simulink model "generic_Truck_And_Trailer"  (R2025a)
settings: Solver=VariableStepAuto  StartTime=0.0  StopTime=350  FixedStep=0.01  MaxStep=0.001  RelTol=1e-3  EnableMultiTasking=on
libraries: TruckMaker4SL x250, simulink x1
(part 9 of 11)

== matlab function generic_Truck_And_Trailer/TruckMaker/Tractor_Subsystem /ONE_TRACK_MODEL_TRACTOR_UKF/MATLAB Function2 ==
  data: z input; u input; Q input; R input; Ts input; xhat output; data input; P output; dxdt output; innovation output; K_out output; S_out output; z_pred_out output
function [xhat, P, dxdt, innovation, K_out, S_out, z_pred_out] = UKF_OneTrack_IMU(z, u, Q, R, Ts, data)
z=z(1:5);
persistent x Pk dxdt_old t

%% =========================
%% INIT
%% =========================
if isempty(x)
    % [vx vy wz Cf Cr bax]
    x = [15;0.1;0.1;7.5;7.5;0];
end

if isempty(Pk)
    Pk = diag([0.1 0.1 0.1 5 5 0.5]);
end

if isempty(dxdt_old)
    dxdt_old = zeros(6,1);
end

if isempty(t)
    t = 0;
end

t = data;

if t < 30
    xhat = x;
    P = Pk;
    dxdt = dxdt_old;
    innovation = zeros(length(z),1);
    K_out = zeros(length(x), length(z));
    S_out = eye(length(z));
    z_pred_out = zeros(length(z),1);
    return
end

IDX_VX = 3;
IDX_VY = 4;

%% =========================
%% VEHICLE CONSTANTS
%% =========================
g  = 9.82;

p_cog = [3.473;0;0.925];
p_fax = [4.520;0;0.490];
p_rax = [0.950;0;0.490];
p_imu = [3.600;0;1.000];

lf = abs(p_fax(1)-p_cog(1));
lr = abs(p_cog(1)-p_rax(1));
L  = lf + lr;
h  = p_cog(3);

Rfax = p_fax - p_cog; Rfax(3) = -p_cog(3);
Rrax = p_rax - p_cog; Rrax(3) = -p_cog(3);
Rcog = p_imu - p_cog;

%% =========================
%% INPUTS
%% =========================
delta = u(1);
T_rl  = u(2);
T_rr  = u(3);
Rwheel = 0.505;
Fx_vehicle = (T_rl + T_rr)/Rwheel;

%% =========================
%% UKF PARAMS
%% =========================
n = length(x);
nSPx = 2*n + 1;

W0 = 1 - n/3;
Wi = (1 - W0)/(2*n);
gamma = sqrt(n/(1-W0));

%% =========================
%% SIGMA POINTS (PRIOR)
%% =========================
Pk = (Pk + Pk')/2 + 1e-9*eye(n);
Sx = chol(Pk,'lower');

X_pre = zeros(n,nSPx);
X_pre(:,1) = x;

for i=1:n
    X_pre(:,i+1)   = x + gamma*Sx(:,i);
    X_pre(:,i+1+n) = x - gamma*Sx(:,i);
end

%% =========================
%% PREDICTION
%% =========================
X_pred = zeros(n,nSPx);
dxdt_model = zeros(n,1);

m = 6800; 
Jz = 12994.917;

for k=1:nSPx

    Xk = X_pre(:,k);

    vx = Xk(1); vy = Xk(2); wz = Xk(3);
    Cf = Xk(4); Cr = Xk(5);
    bax = Xk(6);

    v_cog = [vx; vy; 0]; 
    omega = [0; 0; wz];

    Rotf = [cos(delta) -sin(delta) 0;
            sin(delta)  cos(delta) 0;
            0 0 1];

    vf = Rotf.'*(v_cog + cross(omega,Rfax));
    vr = v_cog + cross(omega,Rrax);

    alpha_f = atan2(vf(2), max(abs(vf(1)),0.1));
    alpha_r = atan2(vr(2), max(abs(vr(1)),0.1));

    ax_est = Fx_vehicle/m + vy*wz;

    Ffz = m*g*lr/L - m*ax_est*h/L;
    Frz = m*g*lf/L + m*ax_est*h/L;

    Fy_f = -Cf*alpha_f*Ffz;
    Fy_r = -Cr*alpha_r*Frz;

    dvx = (Fx_vehicle - Fy_f*sin(delta))/m + vy*wz + bax;

    % Testa DÄMPNING här (NYCKELN!)
    dvy = (Fy_f*cos(delta)+Fy_r)/m - vx*wz;

    dwz = (lf*Fy_f*cos(delta) - lr*Fy_r)/Jz;

    if k==1
        dxdt_model = [dvx; dvy; dwz; 0; 0; 0];
    end

    X_pred(:,k) = [
        vx + Ts*dvx
        vy + Ts*dvy
        wz + Ts*dwz
        Cf
        Cr
        bax
    ];
end

%% =========================
%% MEAN
%% =========================
x_pred = zeros(n,1);
for k=1:nSPx
    w = (k==1)*W0 + (k>1)*Wi;
    x_pred = x_pred + w*X_pred(:,k);
end

%% =========================
%% COVARIANCE
%% =========================
P_pred = zeros(n);
for k=1:nSPx
    w = (k==1)*W0 + (k>1)*Wi;
    dx = X_pred(:,k) - x_pred;
    P_pred = P_pred + w*(dx*dx');
end

P_pred = P_pred + Q*Ts;
P_pred = (P_pred + P_pred')/2 + 1e-9*eye(n);

%% =========================
%% SIGMA POINTS (POST)
%% =========================
Sx = chol(P_pred,'lower');

X_post = zeros(n,nSPx);
X_post(:,1) = x_pred;

for i=1:n
    X_post(:,i+1)   = x_pred + gamma*Sx(:,i);
    X_post(:,i+1+n) = x_pred - gamma*Sx(:,i);
end

%% =========================
%% MEASUREMENT MODEL
%% =========================
Z = zeros(length(z), nSPx);

for k=1:nSPx

    Xk = X_post(:,k);

    vx = Xk(1); vy = Xk(2); wz = Xk(3);
    Cf = Xk(4); Cr = Xk(5);
    bax = Xk(6);

    v_cog = [vx; vy; 0]; 
    omega=[0;0;wz];

    Rotf=[cos(delta) -sin(delta) 0;
          sin(delta)  cos(delta) 0;
          0 0 1];

    vf = Rotf.'*(v_cog+cross(omega,Rfax));
    vr = v_cog+cross(omega,Rrax);

    alpha_f = atan2(vf(2), max(abs(vf(1)),0.1));
    alpha_r = atan2(vr(2), max(abs(vr(1)),0.1));

    ax_est = Fx_vehicle/m + vy*wz;

    Ffz = m*g*lr/L - m*ax_est*h/L;
    Frz = m*g*lf/L + m*ax_est*h/L;

    Fy_f = -Cf*alpha_f*Ffz;
    Fy_r = -Cr*alpha_r*Frz;
    
    dvx = (Fx_vehicle - Fy_f*sin(delta))/m;
    dvy = (Fy_f*cos(delta)+Fy_r)/m;
    dwz = (lf*Fy_f*cos(delta) - lr*Fy_r)/Jz;

    a_cog = [dvx; dvy; 0];
    alpha_vec=[0;0;dwz];

    a_imu = a_cog + cross(omega,cross(omega,Rcog)) + cross(alpha_vec,Rcog);
    v_imu = v_cog + cross(omega,Rcog);

    ax_meas = a_imu(1) + bax;

    Z(:,k) = [
        ax_meas
        a_imu(2)
        v_imu(1:2)
        wz
    ];
end

%% =========================
%% MEASUREMENT MEAN
%% =========================
z_pred = zeros(length(z),1);
for k=1:nSPx
    w = (k==1)*W0 + (k>1)*Wi;
    z_pred = z_pred + w*Z(:,k);
end

%% =========================
%% SENSOR SELECTION
%% =========================
valid_idx = true(length(z),1);

if isnan(z(IDX_VX))
    valid_idx(IDX_VX) = false;
    valid_idx(IDX_VY) = false;
end

valid_idx = valid_idx & ~isnan(z);

z_used = z(valid_idx);
z_pred_used = z_pred(valid_idx);
Z_used = Z(valid_idx,:);
R_used = R(valid_idx,valid_idx);

%% =========================
%% S + Pxz
%% =========================
S_cov = zeros(length(z_used));
Pxz = zeros(n,length(z_used));

for k=1:nSPx
    w = (k==1)*W0 + (k>1)*Wi;

    dz = Z_used(:,k)-z_pred_used;
    dx = X_post(:,k)-x_pred;

    S_cov = S_cov + w*(dz*dz');
    Pxz = Pxz + w*(dx*dz');
end

S_cov = S_cov + R_used;
S_cov = (S_cov + S_cov')/2 + 1e-9*eye(size(S_cov));

%% =========================
%% UPDATE
%% =========================
K = Pxz / S_cov;

x = x_pred + K*(z_used - z_pred_used);
Pk = P_pred - K*S_cov*K';
Pk = (Pk + Pk')/2 + 1e-9*eye(n);

%% =========================
%% OUTPUT
%% =========================
xhat = x;
P = Pk;
dxdt = dxdt_model;

innovation = zeros(length(z),1);
innovation(valid_idx) = z_used - z_pred_used;

K_out = zeros(n,length(z));
K_out(:,valid_idx) = K;

S_out = zeros(length(z));
S_out(valid_idx,valid_idx) = S_cov;

z_pred_out = z_pred;

end

== matlab function generic_Truck_And_Trailer/TruckMaker/Tractor_Subsystem /ONE_TRACK_MODEL_TRACTOR_UKF/UKF_ONE_TRACK1 ==
  data: z input; u input; xhat output; Q input; R input; Ts input; P output; dxdt output; innovation output; K_out output; S_out output; z_pred_out output; data input
function [xhat, P, dxdt, innovation, K_out, S_out, z_pred_out] = UKF_OneTrack_IMU(z, u, Q, R, Ts,data)

persistent x Pk dxdt_old t p_nom Pp

if isempty(x)
    x = [15;0.1;0.1;7.5;7.5];
end
if isempty(Pk)
    Pk = diag([0.1 0.1 0.1 5 5]);
end
if isempty(dxdt_old)
    dxdt_old = zeros(5,1);
end
if isempty(t)
    t = 0;
end
if isempty(p_nom)
    p_nom = [6800; 12994.917];
    Pp = diag([5000, 20000]).^2;
end

T_sim = 0.001;
t = t + T_sim;
t=data;

if t < 30
    xhat = x;
    P = Pk;
    dxdt = dxdt_old;
    innovation = zeros(length(z),1);
    K_out = zeros(length(x), length(z));
    S_out = eye(length(z));
    z_pred_out = zeros(length(z),1);
    return
end

IDX_VX  = 3; 
IDX_WRL = 6; 
IDX_WRR = 7;

g  = 9.82;

p_cog = [3.473;0;0.925];
p_fax = [4.520;0;0.490];
p_rax = [0.950;0;0.490];
p_imu = [3.600;0;1.000];

lf = abs(p_fax(1)-p_cog(1));
lr = abs(p_cog(1)-p_rax(1));
L  = lf + lr;
h  = p_cog(3);

Rfax = p_fax - p_cog; Rfax(3) = -p_cog(3);
Rrax = p_rax - p_cog; Rrax(3) = -p_cog(3);
Rcog = p_imu - p_cog;

delta = u(1);
T_rl  = u(2);
T_rr  = u(3);
Rwheel = 0.505;
Fx_vehicle = (T_rl + T_rr)/Rwheel;

n  = length(x);
np = length(p_nom);
nSPx = 2*n + 1;
nSPp = 2*np;
nSP  = nSPx + nSPp;

W0 = 1 - (n + np)/3;
Wi = (1 - W0)/(2*(n + np));
gamma = sqrt((n + np)/(1 - W0));

%% ===== STATE SIGMA =====
Pk = (Pk + Pk')/2 + 1e-9*eye(n);
Sx = chol(Pk,'lower');

X = zeros(n,nSPx);
X(:,1) = x;
for i=1:n
    X(:,i+1)   = x + gamma*Sx(:,i);
    X(:,i+1+n) = x - gamma*Sx(:,i);
end

%% ===== PARAM SIGMA =====
Pp = (Pp + Pp')/2 + 1e-9*eye(np);
Sp = chol(Pp,'lower');

SPp = zeros(np,nSPp);
for i=1:np
    SPp(:,i)    = p_nom + gamma*Sp(:,i);
    SPp(:,i+np) = p_nom - gamma*Sp(:,i);
end

%% ===== PREDICTION =====
X_prop = zeros(n,nSP);
dxdt_model = zeros(5,1);

for k=1:nSP
    if k <= nSPx
        Xk = X(:,k); 
        pk = p_nom;
    else
        Xk = x; 
        pk = SPp(:,k-nSPx);
    end

    vx=Xk(1); vy=Xk(2); wz=Xk(3); Cf=Xk(4); Cr=Xk(5);
    m=pk(1); Jz=pk(2);

    v_cog=[vx;vy;0]; omega=[0;0;wz];
    Rotf=[cos(delta) -sin(delta) 0; sin(delta) cos(delta) 0; 0 0 1];

    vf=Rotf.'*(v_cog+cross(omega,Rfax));
    vr=v_cog+cross(omega,Rrax);

    alpha_f=atan2(vf(2),max(abs(vf(1)),0.1));
    alpha_r=atan2(vr(2),max(abs(vr(1)),0.1));

    ax_est=Fx_vehicle/m+vy*wz;

    Ffz=m*g*lr/L - m*ax_est*h/L;
    Frz=m*g*lf/L + m*ax_est*h/L;

    Fy_f=-Cf*alpha_f*Ffz;
    Fy_r=-Cr*alpha_r*Frz;

    dvx=(Fx_vehicle - Fy_f*sin(delta))/m + vy*wz;
    dvy=(Fy_f*cos(delta)+Fy_r)/m - vx*wz;
    dwz=(lf*Fy_f*cos(delta) - lr*Fy_r)/Jz;

    if k==1
        dxdt_model=[dvx;dvy;dwz;0;0];
    end

    X_prop(:,k)=[vx+Ts*dvx; vy+Ts*dvy; wz+Ts*dwz; Cf; Cr];
end

%% ===== MEAN =====
x_pred=zeros(n,1);
for k=1:nSP
    w=(k==1)*W0 + (k>1)*Wi;
    x_pred=x_pred + w*X_prop(:,k);
end

%% ===== COV =====
P_pred=zeros(n);
for k=1:nSPx
    w=(k==1)*W0 + (k>1)*Wi;
    dx=X_prop(:,k)-x_pred;
    P_pred=P_pred + w*(dx*dx');
end
P_pred=P_pred + Q*Ts;

%% ===== NEW SIGMA POINTS =====
P_pred=(P_pred+P_pred')/2 + 1e-9*eye(n);
Sx=chol(P_pred,'lower');

SPx_new=zeros(n,nSPx);
SPx_new(:,1)=x_pred;

for i=1:n
    SPx_new(:,i+1)=x_pred+gamma*Sx(:,i);
    SPx_new(:,i+1+n)=x_pred-gamma*Sx(:,i);
end

%% ===== MEASUREMENT =====
Z=zeros(length(z),nSP);

for k=1:nSP
    if k<=nSPx
        Xk=SPx_new(:,k);
        pk=p_nom;
    else
        Xk=x_pred;
        pk=SPp(:,k-nSPx);
    end

    vx=Xk(1); vy=Xk(2); wz=Xk(3);
    Cf=Xk(4); Cr=Xk(5);

    m=pk(1); Jz=pk(2);

    v_cog=[vx;vy;0]; omega=[0;0;wz];
    Rotf=[cos(delta) -sin(delta) 0; sin(delta) cos(delta) 0; 0 0 1];

    vf=Rotf.'*(v_cog+cross(omega,Rfax));
    vr=v_cog+cross(omega,Rrax);

    alpha_f=atan2(vf(2),max(abs(vf(1)),0.1));
    alpha_r=atan2(vr(2),max(abs(vr(1)),0.1));

    ax_est=Fx_vehicle/m+vy*wz;

    Ffz=m*g*lr/L - m*ax_est*h/L;
    Frz=m*g*lf/L + m*ax_est*h/L;

    Fy_f=-Cf*alpha_f*Ffz;
    Fy_r=-Cr*alpha_r*Frz;

    dvx=(Fx_vehicle - Fy_f*sin(delta))/m;
    dvy=(Fy_f*cos(delta)+Fy_r)/m;
    dwz=(lf*Fy_f*cos(delta) - lr*Fy_r)/Jz;

    a_cog=[dvx;dvy;0];
    alpha_vec=[0;0;dwz];

    a_imu=a_cog + cross(omega,cross(omega,Rcog)) + cross(alpha_vec,Rcog);
    v_imu=v_cog + cross(omega,Rcog);

    omega_rl=vx/Rwheel;
    omega_rr=vx/Rwheel;

    Z(:,k)=[a_imu(1:2); v_imu(1:2); wz; omega_rl; omega_rr];
end

%% ===== z mean =====
z_pred=zeros(length(z),1);
for k=1:nSP
    w=(k==1)*W0 + (k>1)*Wi;
    z_pred=z_pred + w*Z(:,k);
end

%% ===== SENSOR SELECTION =====
valid_idx=true(length(z),1);

if ~isnan(z(IDX_VX))
    valid_idx(IDX_WRL)=false;
    valid_idx(IDX_WRR)=false;
else
    valid_idx(IDX_VX)=false;
end

valid_idx=valid_idx & ~isnan(z);

z_used=z(valid_idx);
z_pred_used=z_pred(valid_idx);
Z_used=Z(valid_idx,:);
R_used=R(valid_idx,valid_idx);

%% ===== S =====
S_cov=zeros(length(z_used));
for k=1:nSP
    w=(k==1)*W0 + (k>1)*Wi;
    dz=Z_used(:,k)-z_pred_used;
    S_cov=S_cov + w*(dz*dz');
end

S_cov=S_cov + R_used;
S_cov=(S_cov+S_cov')/2 + 1e-9*eye(size(S_cov));

%% ===== Pxz =====
Pxz=zeros(n,length(z_used));
for k=1:nSPx
    w=(k==1)*W0 + (k>1)*Wi;
    dx=SPx_new(:,k)-x_pred;
    dz=Z_used(:,k)-z_pred_used;
    Pxz=Pxz + w*(dx*dz');
end

%% ===== UPDATE =====
K=Pxz/S_cov;

x=x_pred + K*(z_used - z_pred_used);
Pk=P_pred - K*S_cov*K';
Pk=(Pk+Pk')/2 + 1e-9*eye(n);

%% ===== OUTPUT =====
xhat=x;
P=Pk;
dxdt=dxdt_model;

innovation=zeros(length(z),1);
innovation(valid_idx)=z_used - z_pred_used;

K_out=zeros(n,length(z));
K_out(:,valid_idx)=K;

S_out=zeros(length(z));
S_out(valid_idx,valid_idx)=S_cov;

z_pred_out=z_pred;

end

== matlab function generic_Truck_And_Trailer/TruckMaker/Tractor_Subsystem /ONE_TRACK_MODEL_TRACTOR_UKF/Working Model with 5 measurements  ==
  data: z input; u input; xhat output; Q input; R input; Ts input; P output; dxdt output; innovation output; K_out output; S_out output; z_pred_out output
function [xhat, P, dxdt, innovation, K_out, S_out, z_pred_out] = UKF_OneTrack_IMU(z, u, Q, R, Ts)

% z = [ax; ay; vx; vy; wz]

%% =========================
%% PERSISTENT VARIABLES
%% =========================
persistent x Pk dxdt_old t

if isempty(x)
    x = [15;0.1;0.1;7.5;7.5];   % [vx vy wz Cf Cr]
end
if isempty(Pk)
    Pk = diag([0.1 0.1 0.1 2 2]);
end
if isempty(dxdt_old)
    dxdt_old = zeros(5,1);
end
if isempty(t)
    t = 0;
end

%% =========================
%% TIME UPDATE
%% =========================
t = t + 0.001;

start_time = 30;
if t < start_time
    xhat = x;
    P = Pk;
    dxdt = dxdt_old;

    innovation = zeros(length(z),1);
    K_out = zeros(length(x), length(z));
    S_out = eye(length(z));
    z_pred_out = zeros(length(z),1);
    return
end

%% =========================
%% VEHICLE PARAMETERS
%% =========================
m  = 6800;
g  = 9.82;
Jz = 12994.917;

p_cog = [3.473;0;0.925];
p_fax = [4.520;0;0.490];
p_rax = [0.950;0;0.490];
p_imu = [3.600;0;1.000];

lf = abs(p_fax(1)-p_cog(1));
lr = abs(p_cog(1)-p_rax(1));
L  = lf + lr;
h  = p_cog(3);

Rfax = p_fax - p_cog; Rfax(3) = -p_cog(3);
Rrax = p_rax - p_cog; Rrax(3) = -p_cog(3);
Rcog = p_imu - p_cog;

%% =========================
%% INPUTS
%% =========================
delta = u(1);
T_rl  = u(2);
T_rr  = u(3);
Rwheel = 0.505;

Fx_vehicle = (T_rl + T_rr)/(Rwheel);

%% =========================
%% UKF PARAMETERS
%% =========================
n = length(x);
W0 = 1 - n/3;
Wi = (1 - W0)/(2*n);
gamma = sqrt(n/(1-W0));

Pk = (Pk+Pk')/2 + 1e-9*eye(n);
S = chol(Pk,'lower');

%% =========================
%% SIGMA POINTS
%% =========================
X = zeros(n,2*n+1);
X(:,1) = x;

for i=1:n
    X(:,i+1)   = x + gamma*S(:,i);
    X(:,i+1+n) = x - gamma*S(:,i);
end

%% =========================
%% PREDICTION
%% =========================
X_pred = zeros(n,2*n+1);
dxdt_model = zeros(5,1);

for k=1:2*n+1

    vx = X(1,k);
    vy = X(2,k);
    wz = X(3,k);
    Cf = X(4,k);
    Cr = X(5,k);

    v_cog = [vx;vy;0];
    omega = [0;0;wz];

    Rotf = [cos(delta) -sin(delta) 0;
            sin(delta)  cos(delta) 0;
            0 0 1];

    vf = Rotf.'*(v_cog + cross(omega,Rfax));
    vr = v_cog + cross(omega,Rrax);

    alpha_f = atan2(vf(2), max(abs(vf(1)),0.1));
    alpha_r = atan2(vr(2), max(abs(vr(1)),0.1));

    ax_est = Fx_vehicle/m + vy*wz;

    Ffz = m*g*lr/L - m*ax_est*h/L;
    Frz = m*g*lf/L + m*ax_est*h/L;

    Fy_f = -Cf * alpha_f * Ffz;
    Fy_r = -Cr * alpha_r * Frz;

    dvx = (Fx_vehicle - Fy_f*sin(delta))/m + vy*wz;
    dvy = (Fy_f*cos(delta) + Fy_r)/m - vx*wz;
    dwz = (lf*Fy_f*cos(delta) - lr*Fy_r)/Jz;

    if k==1
        dxdt_model = [dvx; dvy; dwz; 0; 0];
    end

    X_pred(:,k) = [
        vx + Ts*dvx
        vy + Ts*dvy
        wz + Ts*dwz
        Cf
        Cr
    ];
end

%% =========================
%% MEAN + COV
%% =========================
x_pred = W0*X_pred(:,1);
for k=2:2*n+1
    x_pred = x_pred + Wi*X_pred(:,k);
end

P_pred = zeros(n);
for k=1:2*n+1
    w = (k==1)*W0 + (k>1)*Wi;
    dx = X_pred(:,k)-x_pred;
    P_pred = P_pred + w*(dx*dx');
end
P_pred = P_pred + Q*Ts;

%% =========================
%% MEASUREMENT MODEL
%% =========================
Z = zeros(length(z),2*n+1);

for k=1:2*n+1

    vx = X_pred(1,k);
    vy = X_pred(2,k);
    wz = X_pred(3,k);
    Cf = X_pred(4,k);
    Cr = X_pred(5,k);

    v_cog = [vx;vy;0];
    omega = [0;0;wz];

    Rotf = [cos(delta) -sin(delta) 0;
            sin(delta)  cos(delta) 0;
            0 0 1];

    vf = Rotf.'*(v_cog + cross(omega,Rfax));
    vr = v_cog + cross(omega,Rrax);

    alpha_f = atan2(vf(2), max(abs(vf(1)),0.1));
    alpha_r = atan2(vr(2), max(abs(vr(1)),0.1));

    ax_est = Fx_vehicle/m + vy*wz;

    Ffz = m*g*lr/L - m*ax_est*h/L;
    Frz = m*g*lf/L + m*ax_est*h/L;

    Fy_f = -Cf * alpha_f * Ffz;
    Fy_r = -Cr * alpha_r * Frz;

    dvx = (Fx_vehicle - Fy_f*sin(delta))/m;
    dvy = (Fy_f*cos(delta) + Fy_r)/m;
    dwz = (lf*Fy_f*cos(delta) - lr*Fy_r)/Jz;

    a_cog = [dvx; dvy; 0];
    alpha_vec = [0;0;dwz];

    a_imu = a_cog + cross(omega,cross(omega,Rcog)) + cross(alpha_vec,Rcog);
    v_imu = v_cog + cross(omega,Rcog);

    Z(:,k) = [a_imu(1:2); v_imu(1:2); wz];
end

%% =========================
%% HANDLE NaN MEASUREMENTS
%% =========================
valid_idx = ~isnan(z);

z_used      = z(valid_idx);
z_pred      = W0*Z(:,1);
for k=2:2*n+1
    z_pred = z_pred + Wi*Z(:,k);
end

z_pred_used = z_pred(valid_idx);
Z_used      = Z(valid_idx,:);
R_used      = R(valid_idx, valid_idx);

%% =========================
%% S
%% =========================
S_cov = zeros(length(z_used));
for k=1:2*n+1
    w = (k==1)*W0 + (k>1)*Wi;
    dz = Z_used(:,k)-z_pred_used;
    S_cov = S_cov + w*(dz*dz');
end
S_cov = S_cov + R_used;

%% =========================
%% Pxz
%% =========================
Pxz = zeros(n,length(z_used));
for k=1:2*n+1
    w = (k==1)*W0 + (k>1)*Wi;
    dx = X_pred(:,k)-x_pred;
    dz = Z_used(:,k)-z_pred_used;
    Pxz = Pxz + w*(dx*dz');
end

%% =========================
%% UPDATE
%% =========================
K = Pxz / S_cov;

x = x_pred + K*(z_used - z_pred_used);
Pk = P_pred - K*S_cov*K';
Pk = (Pk+Pk')/2 + 1e-9*eye(n);

%% =========================
%% OUTPUTS
%% =========================
dxdt_old = dxdt_model;

xhat = x;
P = Pk;
dxdt = dxdt_old;

innovation = zeros(length(z),1);
innovation(valid_idx) = z_used - z_pred_used;

K_out = zeros(n,length(z));
K_out(:,valid_idx) = K;

S_out = zeros(length(z));
S_out(valid_idx,valid_idx) = S_cov;

z_pred_out = z_pred;

end

== matlab function generic_Truck_And_Trailer/TruckMaker/Tractor_Subsystem /ONE_TRACK_MODEL_TRACTOR_UKF/Working Model with 7 measurements ==
  data: z input; u input; xhat output; Q input; R input; Ts input; P output; dxdt output; innovation output; K_out output; S_out output; z_pred_out output; data input
function [xhat, P, dxdt, innovation, K_out, S_out, z_pred_out] = UKF_OneTrack_IMU(z, u, Q, R, Ts,data)

persistent x Pk dxdt_old t p_nom Pp

if isempty(x)
    x = [15;0.1;0.1;7.5;7.5];
end
if isempty(Pk)
    Pk = diag([0.1 0.1 0.1 5 5]);
end
if isempty(dxdt_old)
    dxdt_old = zeros(5,1);
end
if isempty(t)
    t = 0;
end
if isempty(p_nom)
    p_nom = [6800; 12994.917];
    Pp = diag([5000, 20000]).^2;
end

T_sim = 0.001;
t = t + T_sim;
t=data;

if t < 30
    xhat = x;
    P = Pk;
    dxdt = dxdt_old;
    innovation = zeros(length(z),1);
    K_out = zeros(length(x), length(z));
    S_out = eye(length(z));
    z_pred_out = zeros(length(z),1);
    return
end

IDX_VX  = 3; 
IDX_WRL = 6; 
IDX_WRR = 7;

g  = 9.82;

p_cog = [3.473;0;0.925];
p_fax = [4.520;0;0.490];
p_rax = [0.950;0;0.490];
p_imu = [3.600;0;1.000];

lf = abs(p_fax(1)-p_cog(1));
lr = abs(p_cog(1)-p_rax(1));
L  = lf + lr;
h  = p_cog(3);

Rfax = p_fax - p_cog; Rfax(3) = -p_cog(3);
Rrax = p_rax - p_cog; Rrax(3) = -p_cog(3);
Rcog = p_imu - p_cog;

delta = u(1);
T_rl  = u(2);
T_rr  = u(3);
Rwheel = 0.505;
Fx_vehicle = (T_rl + T_rr)/Rwheel;

n  = length(x);
np = length(p_nom);
nSPx = 2*n + 1;
nSPp = 2*np;
nSP  = nSPx + nSPp;

W0 = 1 - (n + np)/3;
Wi = (1 - W0)/(2*(n + np));
gamma = sqrt((n + np)/(1 - W0));

%% ===== STATE SIGMA =====
Pk = (Pk + Pk')/2 + 1e-9*eye(n);
Sx = chol(Pk,'lower');

X = zeros(n,nSPx);
X(:,1) = x;
for i=1:n
    X(:,i+1)   = x + gamma*Sx(:,i);
    X(:,i+1+n) = x - gamma*Sx(:,i);
end

%% ===== PARAM SIGMA =====
Pp = (Pp + Pp')/2 + 1e-9*eye(np);
Sp = chol(Pp,'lower');

SPp = zeros(np,nSPp);
for i=1:np
    SPp(:,i)    = p_nom + gamma*Sp(:,i);
    SPp(:,i+np) = p_nom - gamma*Sp(:,i);
end

%% ===== PREDICTION =====
X_prop = zeros(n,nSP);
dxdt_model = zeros(5,1);

for k=1:nSP
    if k <= nSPx
        Xk = X(:,k); 
        pk = p_nom;
    else
        Xk = x; 
        pk = SPp(:,k-nSPx);
    end

    vx=Xk(1); vy=Xk(2); wz=Xk(3); Cf=Xk(4); Cr=Xk(5);
    m=pk(1); Jz=pk(2);

    v_cog=[vx;vy;0]; omega=[0;0;wz];
    Rotf=[cos(delta) -sin(delta) 0; sin(delta) cos(delta) 0; 0 0 1];

    vf=Rotf.'*(v_cog+cross(omega,Rfax));
    vr=v_cog+cross(omega,Rrax);

    alpha_f=atan2(vf(2),max(abs(vf(1)),0.1));
    alpha_r=atan2(vr(2),max(abs(vr(1)),0.1));

    ax_est=Fx_vehicle/m+vy*wz;

    Ffz=m*g*lr/L - m*ax_est*h/L;
    Frz=m*g*lf/L + m*ax_est*h/L;

    Fy_f=-Cf*alpha_f*Ffz;
    Fy_r=-Cr*alpha_r*Frz;

    dvx=(Fx_vehicle - Fy_f*sin(delta))/m + vy*wz;
    dvy=(Fy_f*cos(delta)+Fy_r)/m - vx*wz;
    dwz=(lf*Fy_f*cos(delta) - lr*Fy_r)/Jz;

    if k==1
        dxdt_model=[dvx;dvy;dwz;0;0];
    end

    X_prop(:,k)=[vx+Ts*dvx; vy+Ts*dvy; wz+Ts*dwz; Cf; Cr];
end

%% ===== MEAN =====
x_pred=zeros(n,1);
for k=1:nSP
    w=(k==1)*W0 + (k>1)*Wi;
    x_pred=x_pred + w*X_prop(:,k);
end

%% ===== COV =====
P_pred=zeros(n);
for k=1:nSPx
    w=(k==1)*W0 + (k>1)*Wi;
    dx=X_prop(:,k)-x_pred;
    P_pred=P_pred + w*(dx*dx');
end
P_pred=P_pred + Q*Ts;

%% ===== NEW SIGMA POINTS =====
P_pred=(P_pred+P_pred')/2 + 1e-9*eye(n);
Sx=chol(P_pred,'lower');

SPx_new=zeros(n,nSPx);
SPx_new(:,1)=x_pred;

for i=1:n
    SPx_new(:,i+1)=x_pred+gamma*Sx(:,i);
    SPx_new(:,i+1+n)=x_pred-gamma*Sx(:,i);
end

%% ===== MEASUREMENT =====
Z=zeros(length(z),nSP);

for k=1:nSP
    if k<=nSPx
        Xk=SPx_new(:,k);
        pk=p_nom;
    else
        Xk=x_pred;
        pk=SPp(:,k-nSPx);
    end

    vx=Xk(1); vy=Xk(2); wz=Xk(3);
    Cf=Xk(4); Cr=Xk(5);

    m=pk(1); Jz=pk(2);

    v_cog=[vx;vy;0]; omega=[0;0;wz];
    Rotf=[cos(delta) -sin(delta) 0; sin(delta) cos(delta) 0; 0 0 1];

    vf=Rotf.'*(v_cog+cross(omega,Rfax));
    vr=v_cog+cross(omega,Rrax);

    alpha_f=atan2(vf(2),max(abs(vf(1)),0.1));
    alpha_r=atan2(vr(2),max(abs(vr(1)),0.1));

    ax_est=Fx_vehicle/m+vy*wz;

    Ffz=m*g*lr/L - m*ax_est*h/L;
    Frz=m*g*lf/L + m*ax_est*h/L;

    Fy_f=-Cf*alpha_f*Ffz;
    Fy_r=-Cr*alpha_r*Frz;

    dvx=(Fx_vehicle - Fy_f*sin(delta))/m;
    dvy=(Fy_f*cos(delta)+Fy_r)/m;
    dwz=(lf*Fy_f*cos(delta) - lr*Fy_r)/Jz;

    a_cog=[dvx;dvy;0];
    alpha_vec=[0;0;dwz];

    a_imu=a_cog + cross(omega,cross(omega,Rcog)) + cross(alpha_vec,Rcog);
    v_imu=v_cog + cross(omega,Rcog);

    omega_rl=vx/Rwheel;
    omega_rr=vx/Rwheel;

    Z(:,k)=[a_imu(1:2); v_imu(1:2); wz; omega_rl; omega_rr];
end

%% ===== z mean =====
z_pred=zeros(length(z),1);
for k=1:nSP
    w=(k==1)*W0 + (k>1)*Wi;
    z_pred=z_pred + w*Z(:,k);
end

%% ===== SENSOR SELECTION =====
valid_idx=true(length(z),1);

if ~isnan(z(IDX_VX))
    valid_idx(IDX_WRL)=false;
    valid_idx(IDX_WRR)=false;
else
    valid_idx(IDX_VX)=false;
end

valid_idx=valid_idx & ~isnan(z);

z_used=z(valid_idx);
z_pred_used=z_pred(valid_idx);
Z_used=Z(valid_idx,:);
R_used=R(valid_idx,valid_idx);

%% ===== S =====
S_cov=zeros(length(z_used));
for k=1:nSP
    w=(k==1)*W0 + (k>1)*Wi;
    dz=Z_used(:,k)-z_pred_used;
    S_cov=S_cov + w*(dz*dz');
end

S_cov=S_cov + R_used;
S_cov=(S_cov+S_cov')/2 + 1e-9*eye(size(S_cov));

%% ===== Pxz =====
Pxz=zeros(n,length(z_used));
for k=1:nSPx
    w=(k==1)*W0 + (k>1)*Wi;
    dx=SPx_new(:,k)-x_pred;
    dz=Z_used(:,k)-z_pred_used;
    Pxz=Pxz + w*(dx*dz');
end

%% ===== UPDATE =====
K=Pxz/S_cov;

x=x_pred + K*(z_used - z_pred_used);
Pk=P_pred - K*S_cov*K';
Pk=(Pk+Pk')/2 + 1e-9*eye(n);

%% ===== OUTPUT =====
xhat=x;
P=Pk;
dxdt=dxdt_model;

innovation=zeros(length(z),1);
innovation(valid_idx)=z_used - z_pred_used;

K_out=zeros(n,length(z));
K_out(:,valid_idx)=K;

S_out=zeros(length(z));
S_out(valid_idx,valid_idx)=S_cov;

z_pred_out=z_pred;

end

== matlab function generic_Truck_And_Trailer/TruckMaker/Tractor_Subsystem /Subsystem/Ackerman Angle/MATLAB Function ==
  data: delta_l input; delta output; delta_r input
function delta = ackerman_angle(delta_l, delta_r)

delta = acot((cot(delta_l) + cot(delta_r))/2);

end

== matlab function generic_Truck_And_Trailer/TruckMaker/Tractor_Subsystem /Subsystem_Noisey Measurements/MATLAB Function ==
  data: gyro_true input; gyro_meas output
function gyro_meas = imu_gyro_noise(gyro_true)

Fs = 1000;   % sample rate

[meas, ~] = GyroNoise(gyro_true', Fs);

gyro_meas = meas';

end

== matlab function generic_Truck_And_Trailer/TruckMaker/Tractor_Subsystem /Subsystem_Noisey Measurements/MATLAB Function1 ==
  data: acc_true input; acc_meas output
function acc_meas = AccelNoiseBlock(acc_true)

Fs = 1000;

truth = acc_true;      % 1×3

[meas,~] = AccelNoise(truth,Fs);

acc_meas = meas;       % 3×1

end

== matlab function generic_Truck_And_Trailer/TruckMaker/Tractor_Subsystem /Subsystem_Noisey Measurements/MATLAB Function2 ==
  data: truth input; vel_meas output
function vel_meas = imu_vel_noise(truth)
    

sigma = 0.05; % m/s^2 (tune later)

vel_meas = truth + sigma * randn(size(truth));


end

== matlab function generic_Truck_And_Trailer/TruckMaker/Tractor_Subsystem /Subsystem_Noisey Measurements _NAN/MATLAB Function3 ==
  data: truth input; vel_meas output
function vel_meas = imu_vel_noise(truth)
    

sigma = 0.05; % m/s^2 (tune later)

vel_meas = truth + sigma * randn(size(truth));


end

== matlab function generic_Truck_And_Trailer/TruckMaker/Tractor_Subsystem /Subsystem_Noisey Measurements _NAN/MATLAB Function ==
  data: gyro_true input; gyro_meas output
function gyro_meas = imu_gyro_noise(gyro_true)

Fs = 1000;   % sample rate

[meas, ~] = GyroNoise(gyro_true', Fs);

gyro_meas = meas';

end

== matlab function generic_Truck_And_Trailer/TruckMaker/Tractor_Subsystem /Subsystem_Noisey Measurements _NAN/MATLAB Function1 ==
  data: acc_true input; acc_meas output
function acc_meas = AccelNoiseBlock(acc_true)

Fs = 1000;

truth = acc_true;      % 1×3

[meas,~] = AccelNoise(truth,Fs);

acc_meas = meas;       % 3×1

end

== matlab function generic_Truck_And_Trailer/TruckMaker/Tractor_Subsystem /Subsystem_Noisey Measurements _NAN/MATLAB Function2 ==
  data: truth input; vel_meas output
function vel_meas = imu_vel_noise(truth)
    

sigma = 0.05; % m/s^2 (tune later)

vel_meas = truth + sigma * randn(size(truth));


end

== matlab function generic_Truck_And_Trailer/TruckMaker/Tractor_Subsystem /Subsystem_Noisey Measurements/MATLAB Function3 ==
  data: truth input; vel_meas output
function vel_meas = imu_vel_noise(truth)
    

sigma = 0.05; % m/s^2 (tune later)

vel_meas = truth + sigma * randn(size(truth));


end

== matlab function generic_Truck_And_Trailer/TruckMaker/Subsystem1/ONE_TRACK_MODEL_TRACTOR_UKF/TEST_Algorithm  ==
  data: z input; u input; xhat output; Q input; R input; Ts input; data input; P output; dxdt output; innovation output; K_out output; S_out output; z_pred_out output
function [xhat, P, dxdt, innovation, K_out, S_out, z_pred_out] = UKF_TruckTrailer(z,u,Q,R,Ts,data)

persistent x Pk dxdt_old t

%% =========================
%% INIT
%% =========================
if isempty(x)
    x = [15;0.1;0.1;7.5;7.5;0;0;6]; % [vx vy wz Cf Cr psi wz_tr Cr_tr]
end

if isempty(Pk)
    Pk = diag([0.1 0.1 0.1 5 5 0.03 0.1 5]);
end

if isempty(dxdt_old)
    dxdt_old = zeros(8,1);
end

if isempty(t)
    t = 0;
end

t = data;
if t < 30
    xhat=x; P=Pk; dxdt=dxdt_old;
    
    innovation=zeros(length(z),1);
    K_out=zeros(length(x), length(z));
    S_out=eye(length(z));
    z_pred_out=zeros(length(z),1);
    return
end

%% =========================
%% CONSTANTS
%% =========================
g = 9.82;

% Truck
m = 6800; 
Jz = 12994.917; 
Rwheel = 0.49;

w_track = 2.1; % FIXED: Lade till spårvidd för att kunna differentiera hjulhastigheter

% Trailer
m_tr = 31960;
Jz_tr = 145971.764;

% Geometry &  koordinat punkter på Truck
p_cog = [3.473;0;0.925];

p_fax = [4.520;0;0.490];
p_rax = [0.950;0;0.490];
p_imu = [3.600;0;1.000];
hitch = [1.9;0;1.21];
Rcog = p_imu - p_cog;

% Geometry Trailer
p_cog_tr = [-6.195;0;1.95];
p_rax_tr = [-9.0;0;0.490];
hitch_tr = [-1.25;0;1.25];

lf = abs(p_fax(1)-p_cog(1)); 
lr = abs(p_cog(1)-p_rax(1)); 
L = lf + lr;
h = p_cog(3);

Rfax = p_fax - p_cog; Rfax(3)=-p_cog(3);
Rrax = p_rax - p_cog; Rrax(3)=-p_cog(3);
Rhitch = hitch - p_cog;
lhitch = Rhitch(1);

lfhitch = abs(p_fax(1) -hitch(1)); 
lf_tr = abs(hitch_tr(1)-p_cog_tr(1));
lr_tr = abs(p_cog_tr(1)-p_rax_tr(1));
L_tr = lf_tr + lr_tr;
h_tr = p_cog_tr(3);
hHitch= hitch(3);
Rrax_tr = p_rax_tr - hitch_tr; Rrax_tr(3)=-hitch_tr(3);

%% =========================
%% INPUTS
%% =========================
delta = u(1); % steering to road angle 
% Rear wheel drive
T_rl = u(2);   
T_rr = u(3);

Fxh = u(4); %  detta är kraft på dragkrok uttryckt i släpets koordinatsystem
Fyh = u(5); 

% Använder abs() ifall insignalen skulle fluktuera mellan positiv/negativ
Fx_f_brake  = -abs(u(6)) / Rwheel; 
Fx_r_brake  = -abs(u(7)) / Rwheel;
Fx_tr_brake = -abs(u(8)) / Rwheel;

Fx_vehicle = (T_rl+T_rr)/Rwheel + Fx_r_brake +Fx_f_brake + Fx_tr_brake;

%% =========================
%% UKF PARAMS
%% =========================
n = length(x);
nSPx = 2*n+1;
W0 = 1 - n/3;
Wi = (1 - W0)/(2*n);
gamma = sqrt(n/(1 - W0));

%% =========================
%% SIGMA POINTS (PRIOR)
%% =========================
Pk = (Pk+Pk')/2 + 1e-9*eye(n);
Sx = chol(Pk,'lower');
X_pre = zeros(n,nSPx);
X_pre(:,1) = x;
for i=1:n
    X_pre(:,i+1)   = x + gamma*Sx(:,i);
    X_pre(:,i+1+n) = x - gamma*Sx(:,i);
end

%% =========================
%% PREDICTION
%% =========================
X_pred = zeros(n,nSPx);
dxdt_model = zeros(n,1);
for k=1:nSPx
    Xk = X_pre(:,k);
    
    % Traktor CoG
    vx=Xk(1); vy=Xk(2); wz=Xk(3);Cf=Xk(4); Cr=Xk(5);
    
    % Trailer 
    psi=Xk(6); wz_tr=Xk(7); Cr_tr=Xk(8);
    
    v_cog=[vx;vy;0];
    omega=[0;0;wz];
    
    %% ===== TRAILER =====
    v_hitch_truck = v_cog + cross(omega,Rhitch);
    
    Rot_tr=[cos(psi) -sin(psi) 0;
            sin(psi)  cos(psi) 0;
            0 0 1];
    
    omega_tr=[0;0;wz_tr];
    
    % FIXED: Tog bort minustecknet framför Rot_tr för konsekvens
    v_hitch_trailer = Rot_tr.' * v_hitch_truck; 
    
    % velocity of trailer wheel at rear axle contact point  
    v_tr_ax = v_hitch_trailer + cross(omega_tr,Rrax_tr);
    
    % slip
    alpha_tr = atan2(v_tr_ax(2),max(abs(v_tr_ax(1)),0.1));
    
    % load transfer approximation 
    ax_tr = Fxh/m_tr;
    
    % FIXED: Ändrade till minustecken eftersom acceleration flyttar vikten bakåt från dragkroken
    Fz_hitch = m_tr*g*lr_tr/L_tr - m_tr*ax_tr*(h_tr-hHitch)/L_tr;
    Fz_tr    = m_tr*g - Fz_hitch;
    
    % Brush Model 
    Fy_tr = -Cr_tr*alpha_tr*Fz_tr;
    
    %% ===== TRUCK =====
    % Rotation Matris 
    Rotf=[cos(delta) -sin(delta) 0;
          sin(delta)  cos(delta) 0;
          0                0     1];
    
    % velocities at contact point 
    vf = Rotf.'*(v_cog + cross(omega,Rfax));
    vr = v_cog + cross(omega,Rrax);
    
    % slip per wheel 
    alpha_f = atan2(vf(2),max(abs(vf(1)),0.1));
    alpha_r = atan2(vr(2),max(abs(vr(1)),0.1));
    
    F_hitch_trailer=[u(4);u(5);0];
    F_hitch_body= Rot_tr * F_hitch_trailer;
    
    % load transfer approximation
    ax_est = (Fx_vehicle - F_hitch_body(1))/m; % Använder förenklad acceleration utan coriolis för lastöverföring
    
    % FIXED: Exakt momentbalans för Ffz och Frz. Tar hänsyn till var dragkroken faktiskt sitter.
    Ffz = (m*g*lr - m*ax_est*h + Fz_hitch*(hitch(1) - p_rax(1)) - F_hitch_body(1)*hHitch) / L;
    Frz = (m*g*lf + m*ax_est*h + Fz_hitch*(p_fax(1) - hitch(1)) + F_hitch_body(1)*hHitch) / L;
    
    % Säkerhetsspärr mot negativ normalkraft i extrema transienter
    %Ffz = max(Ffz, 100);
    %Frz = max(Frz, 100);

    % brush model 
    Fy_f = -Cf*alpha_f*Ffz;
    Fy_r = -Cr*alpha_r*Frz;
    
    %% ===== DYNAMICS =====
    dvx = (Fx_vehicle - Fy_f*sin(delta) - F_hitch_body(1))/m + vy*wz;
    dvy = (Fy_f*cos(delta) + Fy_r - F_hitch_body(2))/m - vx*wz;
    
    % FIXED: Återinförde dragkrokens sidokraft i lastbilens gir-ekvation
    dwz = (lf*Fy_f*cos(delta) - lr*Fy_r - lhitch*(F_hitch_body(2)))/Jz;
    
    dpsi = wz_tr - wz; % Articulation angle 
    dwz_tr =(-lr_tr*Fy_tr + lf_tr*Fyh)/Jz_tr;
    
    if k==1
        dxdt_model=[dvx;dvy;dwz;0;0;dpsi;dwz_tr;0];
    end
    
    X_pred(:,k) = Xk + Ts*[dvx;
                           dvy;
                           dwz;
                           0;
                           0;
                           dpsi;
                           dwz_tr;
                           0];
end

%% ===== MEAN & COV
x_pred=zeros(n,1);
P_pred=zeros(n);
for k=1:nSPx
    w=(k==1)*W0+(k>1)*Wi;
    x_pred=x_pred+w*X_pred(:,k);
end
for k=1:nSPx
    w=(k==1)*W0+(k>1)*Wi;
    dx=X_pred(:,k)-x_pred;
    P_pred=P_pred+w*(dx*dx');
end
P_pred=P_pred+Q*Ts;
P_pred=(P_pred+P_pred')/2 + 1e-9*eye(n);

%% =========================
%% MEASUREMENT
%% =========================
Sx=chol(P_pred,'lower');
X_post=zeros(n,nSPx);
X_post(:,1)=x_pred;
for i=1:n
    X_post(:,i+1)  =x_pred + gamma*Sx(:,i);
    X_post(:,i+1+n)=x_pred - gamma*Sx(:,i);
end

Z=zeros(length(z),nSPx);
for k=1:nSPx
    Xk=X_post(:,k);
    
    % Traktor CoG
    vx=Xk(1); vy=Xk(2); wz=Xk(3);
    Cf=Xk(4); Cr=Xk(5);
    
    % Trailer 
    psi=Xk(6); wz_tr=Xk(7); Cr_tr=Xk(8); 
    
    v_cog=[vx;vy;0];
    omega=[0;0;wz];
    
    %% ===== TRAILER =====
    v_hitch_truck = v_cog + cross(omega,Rhitch);
    Rot_tr=[cos(psi) -sin(psi) 0;
            sin(psi)  cos(psi) 0;
            0 0 1];
    omega_tr=[0;0;wz_tr];
    
    v_hitch_trailer = Rot_tr.' * v_hitch_truck;
    
    v_tr_ax = v_hitch_trailer + cross(omega_tr,Rrax_tr);
    alpha_tr = atan2(v_tr_ax(2),max(abs(v_tr_ax(1)),0.1));
    
    ax_tr = Fxh / m_tr; 
    
    % FIXED: Ändrade till minustecken
    Fz_hitch = m_tr*g*lr_tr/L_tr - m_tr*ax_tr*(h_tr-hHitch)/L_tr;
    Fz_tr = m_tr*g - Fz_hitch;
    
    Fy_tr = -Cr_tr*alpha_tr*Fz_tr;
    
    %% ===== TRUCK =====    
    Rotf=[cos(delta) -sin(delta) 0;
          sin(delta)  cos(delta) 0;
          0                0     1];
    
    vf = Rotf.'*(v_cog + cross(omega,Rfax));
    vr = v_cog + cross(omega,Rrax);
    
    alpha_f = atan2(vf(2),max(abs(vf(1)),0.1));
    alpha_r = atan2(vr(2),max(abs(vr(1)),0.1));
    
    F_hitch_trailer=[u(4);u(5);0];
    
    F_hitch_body= Rot_tr* F_hitch_trailer;
    
    ax_est = (Fx_vehicle - F_hitch_body(1))/m;
    
    % FIXED: Samma exakta momentbalans som i prediktionsloopen
    Ffz = (m*g*lr - m*ax_est*h + Fz_hitch*(hitch(1) - p_rax(1)) - F_hitch_body(1)*hHitch) / L;
    Frz = (m*g*lf + m*ax_est*h + Fz_hitch*(p_fax(1) - hitch(1)) + F_hitch_body(1)*hHitch) / L;
    
    %Ffz = max(Ffz, 100);
    %Frz = max(Frz, 100);
    
    Fy_f = -Cf*alpha_f*Ffz;
    Fy_r = -Cr*alpha_r*Frz;
    
    %% ===== DYNAMICS (for sensors) =====
    % FIXED: Döpte om dessa till a_specific_x/y för att inte blanda ihop med tillståndsderivatan
    % En IMU mäter inte coriolis, därav ingen vy*wz term här
    a_specific_x = (Fx_vehicle - Fy_f*sin(delta) - F_hitch_body(1))/m;
    a_specific_y = (Fy_f*cos(delta) + Fy_r - F_hitch_body(2))/m;
    
    % Återinförde släpets moment
    dwz = (lf*Fy_f*cos(delta) - lr*Fy_r - lhitch*(F_hitch_body(2)))/Jz;
    
    a_cog = [a_specific_x; a_specific_y; 0];
    alpha_vec = [0; 0; dwz];
    
    a_imu = a_cog + cross(omega,cross(omega,Rcog)) + cross(alpha_vec,Rcog);
    v_imu = v_cog + cross(omega,Rcog);
    
    % FIXED: Lade till spårvidd för att få korrekta differenser vid svängning
    omega_rl = (vx - wz * w_track/2) / Rwheel;
    omega_rr = (vx + wz * w_track/2) / Rwheel;
    omega_tr_ML = (v_tr_ax(1) - wz_tr * w_track/2) / Rwheel;
    omega_tr_MR = (v_tr_ax(1) + wz_tr * w_track/2) / Rwheel;
    
    Z(:,k)=[a_imu(1:2); v_imu(1); v_imu(2); wz; omega_rl; omega_rr; omega_tr_ML; omega_tr_MR];
end

%% ===== REST (sensor selection + update) =====
z_pred=zeros(length(z),1);
for k=1:nSPx
    w=(k==1)*W0+(k>1)*Wi;
    z_pred=z_pred+w*Z(:,k);
end

valid_idx=true(length(z),1);
valid_idx=valid_idx & ~isnan(z);
z_used=z(valid_idx);
z_pred_used=z_pred(valid_idx);
Z_used=Z(valid_idx,:);
R_used=R(valid_idx,valid_idx);

S_cov=zeros(length(z_used));
Pxz=zeros(n,length(z_used));
for k=1:nSPx
    w=(k==1)*W0+(k>1)*Wi;
    dz=Z_used(:,k)-z_pred_used;
    dx=X_post(:,k)-x_pred;
    S_cov=S_cov+w*(dz*dz');
    Pxz=Pxz+w*(dx*dz');
end

S_cov=S_cov+R_used;
S_cov=(S_cov+S_cov')/2 + 1e-9*eye(size(S_cov));
K=Pxz/S_cov;

x=x_pred + K*(z_used - z_pred_used);
Pk=P_pred - K*S_cov*K';
Pk=(Pk+Pk')/2 + 1e-9*eye(n);

%% OUTPUT
xhat=x;
P=Pk;
dxdt=dxdt_model;

innovation=zeros(length(z),1);
innovation(valid_idx)=z_used - z_pred_used;
K_out=zeros(n,length(z));
K_out(:,valid_idx)=K;
S_out=zeros(length(z));
S_out(valid_idx,valid_idx)=S_cov;
z_pred_out=z_pred;

end

== matlab function generic_Truck_And_Trailer/TruckMaker/Subsystem1/Subsystem_Noisey Measurements _NAN/MATLAB Function4 ==
  data: truth input; vel_meas output
function vel_meas = imu_vel_noise(truth)
    

sigma = 0.05; % m/s^2 (tune later)

vel_meas = truth + sigma * randn(size(truth));


end

== matlab function generic_Truck_And_Trailer/TruckMaker/Subsystem1/ONE_TRACK_MODEL_TRACTOR_UKF/UKF_ONE_TRACK2 ==
  data: z input; u input; xhat output; Q input; R input; Ts input; P output; dxdt output; innovation output; K_out output; S_out output; z_pred_out output; data input
function [xhat, P, dxdt, innovation, K_out, S_out, z_pred_out] = UKF_TruckTrailer(z,u,Q,R,Ts,data)
persistent x Pk dxdt_old t Cr_tr_filt
%% =========================
%% INIT
%% =========================
if isempty(x)
    x = [15;0.1;0.1;7.5;7.5;0;0;6]; % [vx vy wz Cf Cr psi wz_tr Cr_tr]
end
if isempty(Pk)
    Pk = diag([0.1 0.1 0.1 5 5 0.03 0.1 5]);
end
if isempty(dxdt_old)
    dxdt_old = zeros(8,1);
end
if isempty(t)
    t = 0;
end

% <-- LÄGG TILL INITIALISERING AV Cr_tr_filt här
if isempty(Cr_tr_filt)
    Cr_tr_filt = 6;  % Startvärde för filtret
end

t = data;
if t < 30
    xhat=x; P=Pk; dxdt=dxdt_old;
    
    innovation=zeros(length(z),1);
    K_out=zeros(length(x), length(z));
    S_out=eye(length(z));
    z_pred_out=zeros(length(z),1);
    return
end
%% =========================
%% CONSTANTS
%% =========================
g = 9.82;
% Truck
m = 6800; 
Jz = 12994.917; 
Rwheel = 0.49;
w_track = 2.1; 
% Trailer
m_tr  = 10350.00;%031960;
Jz_tr = 48289.836;%145971.764;
% Geometry & koordinat punkter på Truck
p_cog = [3.473;0;0.925];
p_fax = [4.520;0;0.490];
p_rax = [0.950;0;0.490];
p_imu = [3.600;0;1.000];
hitch = [1.9;0;1.21];
Rcog = p_imu - p_cog;
% Geometry Trailer
%p_cog_tr = [-6.195;0;1.95];
p_cog_tr = [-6.198;0;1.949];
p_rax_tr = [-9.0;0;0.490];
%hitch_tr = [-1.25;0;1.25];
hitch_tr = [-1.25;0;1.15];
lf = abs(p_fax(1)-p_cog(1)); 
lr = abs(p_cog(1)-p_rax(1)); 
L = lf + lr;
h = p_cog(3);
Rfax = p_fax - p_cog; Rfax(3)=-p_cog(3);
Rrax = p_rax - p_cog; Rrax(3)=-p_cog(3);
Rhitch = hitch - p_cog;
lhitch = Rhitch(1);
lfhitch = abs(p_fax(1) -hitch(1)); 
lf_tr = abs(hitch_tr(1)-p_cog_tr(1));
lr_tr = abs(p_cog_tr(1)-p_rax_tr(1));
L_tr = lf_tr + lr_tr;
h_tr = p_cog_tr(3);
hHitch= hitch(3);
Rrax_tr = p_rax_tr - hitch_tr; Rrax_tr(3)=-hitch_tr(3);
%% =========================
%% INPUTS
%% =========================
delta = u(1); 
T_rl = u(2);   
T_rr = u(3);
Fxh = u(4); 
%Fyh = u(5)*0; 
Fx_f_brake  = -abs(u(6)) / Rwheel; 
Fx_r_brake  = -abs(u(7)) / Rwheel;
%Fx_tr_brake = -abs(u(8)) / Rwheel;
Fx_vehicle = (T_rl+T_rr)/Rwheel + Fx_r_brake +Fx_f_brake;
%% =========================
%% UKF PARAMS
%% =========================
n = length(x);
nSPx = 2*n+1;
W0 = 1 - n/3;
Wi = (1 - W0)/(2*n);
gamma = sqrt(n/(1 - W0));
%% =========================
%% SIGMA POINTS (PRIOR)
%% =========================
Pk = (Pk+Pk')/2 + 1e-9*eye(n);
Sx = chol(Pk,'lower');
X_pre = zeros(n,nSPx);
X_pre(:,1) = x;
for i=1:n
    X_pre(:,i+1)   = x + gamma*Sx(:,i);
    X_pre(:,i+1+n) = x - gamma*Sx(:,i);
end
%% =========================
%% PREDICTION
%% =========================
X_pred = zeros(n,nSPx);
dxdt_model = zeros(n,1);
for k=1:nSPx
    Xk = X_pre(:,k);
    vx=Xk(1); vy=Xk(2); wz=Xk(3);Cf=Xk(4); Cr=Xk(5);
    psi=Xk(6); wz_tr=Xk(7); Cr_tr=Xk(8);
    
    v_cog=[vx;vy;0];
    omega=[0;0;wz];
    
    %% ===== TRAILER =====
    v_hitch_truck = v_cog + cross(omega,Rhitch);
    
    Rot_tr=[cos(psi) -sin(psi) 0;
            sin(psi) cos(psi)  0;
              0           0    1];

    omega_tr=[0;0;wz_tr];
    
    v_hitch_trailer = Rot_tr'  * v_hitch_truck; 
    
    v_tr_ax = v_hitch_trailer + cross(omega_tr,Rrax_tr);
    
    alpha_tr = atan2(v_tr_ax(2),max(abs(v_tr_ax(1)),0.1));
    
    ax_tr = Fxh/m_tr;
    
    Fz_hitch = m_tr*g*lr_tr/L_tr - m_tr*ax_tr*(h_tr-hHitch)/L_tr;
    
    Fz_tr    =  m_tr*g -  Fz_hitch;
    
    Fy_tr = -Cr_tr*alpha_tr*Fz_tr;
    
    % Beräknar modellens sidkraft för hitch
    Fyh_mod = (lr_tr * Fy_tr) / lf_tr; 

    %% ===== TRUCK =====
    Rotf=[cos(delta) -sin(delta) 0;
          sin(delta) cos(delta)  0; 
              0            0     1];

    vf = Rotf.'*(v_cog + cross(omega,Rfax));
    vr = v_cog + cross(omega,Rrax);
    
    alpha_f = atan2(vf(2),max(abs(vf(1)),0.1));
    alpha_r = atan2(vr(2),max(abs(vr(1)),0.1));
    
    F_hitch_trailer=[u(4); Fyh_mod; 0];
    F_hitch_body= Rot_tr * F_hitch_trailer;

    ax_est = (Fx_vehicle - F_hitch_body(1))/m; 
    
    %Ffz = (m*g*lr - m*ax_est*(h-hHitch) + Fz_hitch*(hitch(1) - p_rax(1)) ) / L; %- F_hitch_body(1)*hHitch
    %Frz = (m*g*lf + m*ax_est*(h-hHitch) + Fz_hitch*(p_fax(1) - hitch(1)) ) / L; %+ F_hitch_body(1)*hHitch
    
    Ffz = (m*g*lr - m*ax_est*h + Fz_hitch*(hitch(1) - p_rax(1)) - F_hitch_body(1)*hHitch) / L;
    Frz = (m*g*lf + m*ax_est*h + Fz_hitch*(p_fax(1) - hitch(1)) + F_hitch_body(1)*hHitch) / L;

    Fy_f = -Cf*alpha_f*Ffz;
    Fy_r = -Cr*alpha_r*Frz;
    
    %% ===== DYNAMICS =====
    dvx = (Fx_vehicle - Fy_f*sin(delta) - F_hitch_body(1))/m + vy*wz;
    dvy = (Fy_f*cos(delta) + Fy_r - F_hitch_body(2))/m - vx*wz;
    dwz = (lf*Fy_f*cos(delta) - lr*Fy_r - lhitch*(F_hitch_body(2)))/Jz;
    dpsi = wz - wz_tr; 
    dwz_tr =(lf_tr*Fyh_mod -lr_tr*Fy_tr)/Jz_tr;
    
    if k==1
        dxdt_model=[dvx;dvy;dwz;0;0;dpsi;dwz_tr;0];
    end
    X_pred(:,k) = Xk + Ts*[dvx; dvy; dwz; 0; 0; dpsi; dwz_tr; 0];
end
%% ===== MEAN & COV
x_pred=zeros(n,1);
P_pred=zeros(n);
for k=1:nSPx
    w=(k==1)*W0+(k>1)*Wi;
    x_pred=x_pred+w*X_pred(:,k);
end
for k=1:nSPx
    w=(k==1)*W0+(k>1)*Wi;
    dx=X_pred(:,k)-x_pred;
    P_pred=P_pred+w*(dx*dx');
end
P_pred=P_pred+Q*Ts;
%% =========================
%% MEASUREMENT
%% =========================
Sx=chol((P_pred+P_pred')/2 + 1e-9*eye(n),'lower');
X_post=zeros(n,nSPx);
X_post(:,1)=x_pred;
for i=1:n
    X_post(:,i+1)  =x_pred + gamma*Sx(:,i);
    X_post(:,i+1+n)=x_pred - gamma*Sx(:,i);
end
Z=zeros(10,nSPx); % Fixat till 10 rader
for k=1:nSPx
    Xk=X_post(:,k);
    vx=Xk(1); vy=Xk(2); wz=Xk(3); Cf=Xk(4); Cr=Xk(5);
    psi=Xk(6); wz_tr=Xk(7); Cr_tr=Xk(8); 
    
    v_cog=[vx;vy;0]; omega=[0;0;wz];
    Rot_tr=[cos(psi) -sin(psi) 0;
            sin(psi)  cos(psi) 0;  
                0         0    1];
    omega_tr=[0;0;wz_tr];

    v_hitch_tr = Rot_tr.'  * (v_cog + cross(omega,Rhitch));
    v_tr_ax = v_hitch_tr + cross(omega_tr,Rrax_tr);
    alpha_tr = atan2(v_tr_ax(2),max(abs(v_tr_ax(1)),0.1));
    ax_tr = Fxh / m_tr; 
    
    Fz_hitch = m_tr*g*lr_tr/L_tr - m_tr*ax_tr*(h_tr-hHitch)/L_tr;
    Fy_tr = -Cr_tr*alpha_tr*(m_tr*g - Fz_hitch);
    Fyh_mod = (lr_tr * Fy_tr) / lf_tr; 

    Rotf=[cos(delta) -sin(delta) 0; 
          sin(delta)  cos(delta) 0; 
              0           0      1];
    vf = Rotf.'*(v_cog + cross(omega,Rfax));
    alpha_f = atan2(vf(2),max(abs(vf(1)),0.1));
    alpha_r = atan2(vy - lr*wz, max(abs(vx),0.1));
    
    F_hitch_body= Rot_tr* [u(4); Fyh_mod; 0];
    ax_est = (Fx_vehicle - F_hitch_body(1))/m;
    %Ffz = (m*g*lr - m*ax_est*(h-hHitch) + Fz_hitch*(hitch(1) - p_rax(1)) ) / L; %- F_hitch_body(1)*hHitch
    %Frz = (m*g*lf + m*ax_est*(h-hHitch) + Fz_hitch*(p_fax(1) - hitch(1)) ) / L; %+ F_hitch_body(1)*hHitch

    Ffz = (m*g*lr - m*ax_est*h + Fz_hitch*(hitch(1) - p_rax(1)) - F_hitch_body(1)*hHitch) / L;
    Frz = (m*g*lf + m*ax_est*h + Fz_hitch*(p_fax(1) - hitch(1)) + F_hitch_body(1)*hHitch) / L;
    
    Fy_f = -Cf*alpha_f*Ffz;
    Fy_r = -Cr*alpha_r*Frz;
    
    a_spec_x = (Fx_vehicle - Fy_f*sin(delta) - F_hitch_body(1))/m;
    
    a_spec_y = (Fy_f*cos(delta) + Fy_r - F_hitch_body(2))/m;
    
    dwz = (lf*Fy_f*cos(delta) - lr*Fy_r - lhitch*(F_hitch_body(2)))/Jz;
    
    a_imu = [a_spec_x; a_spec_y; 0] + cross(omega,cross(omega,Rcog)) + cross([0;0;dwz],Rcog);
    v_imu = v_cog + cross(omega,Rcog);
    
    omega_rl = (vx - wz * w_track/2) / Rwheel;
    omega_rr = (vx + wz * w_track/2) / Rwheel;
    omega_tr_ML = (v_tr_ax(1) - wz_tr * w_track/2) / Rwheel;
    omega_tr_MR = (v_tr_ax(1) + wz_tr * w_track/2) / Rwheel;
    
    % Z: [ax; ay; vx; vy; wz; w_rl; w_rr; w_tr_l; w_tr_r; Fyh]
    Z(:,k)=[a_imu(1:2); v_imu(1); v_imu(2); wz; omega_rl; omega_rr; omega_tr_ML; omega_tr_MR; Fyh_mod];
end
%% ===== REST
z_pred=zeros(10,1);
for k=1:nSPx
    w=(k==1)*W0+(k>1)*Wi;
    z_pred=z_pred+w*Z(:,k);
end
valid_idx=true(10,1);
valid_idx=valid_idx & ~isnan(z);
z_used=z(valid_idx);
z_pred_used=z_pred(valid_idx);
Z_used=Z(valid_idx,:);
R_used=R(valid_idx,valid_idx);
S_cov=zeros(length(z_used));
Pxz=zeros(n,length(z_used));
for k=1:nSPx
    w=(k==1)*W0+(k>1)*Wi;
    dz=Z_used(:,k)-z_pred_used;
    dx=X_post(:,k)-x_pred;
    S_cov=S_cov+w*(dz*dz');
    Pxz=Pxz+w*(dx*dz');
end
S_cov=S_cov+R_used;
K=Pxz/S_cov;
x=x_pred + K*(z_used - z_pred_used);
Pk=P_pred - K*S_cov*K';
Pk=(Pk+Pk')/2 + 1e-9*eye(n);


%% ===== EXTRA STABILISERING FÖR Cr_tr =====
% % Begränsa till fysiskt intervall (typiskt 3-20 för trailer)
% x(8) = max(3, min(20, x(8)));
% 
% % Lågpassfilter för att dämpa oscillationer
% % Cr_tr_filt är redan deklarerad som persistent i början
% Cr_tr_filt = 0.95*Cr_tr_filt + 0.05 * x(8);
% x(8) = Cr_tr_filt;
% 
% % Justera process noise - Cr_tr ändras långsamt
% Q(8,8) = 1e-9;
%% OUTPUT
xhat=x;
P=Pk;
dxdt=dxdt_model;

innovation=zeros(length(z),1);
innovation(valid_idx)=z_used - z_pred_used;
K_out=zeros(n,length(z));
K_out(:,valid_idx)=K;
S_out=zeros(length(z));
S_out(valid_idx,valid_idx)=S_cov;
z_pred_out=z_pred;
end
